simulink model "sim_1_twolink_planar_model"  (R2021a)
settings: Solver=ode15s  StartTime=0.0  StopTime=50  RelTol=1e-5  EnableMultiTasking=on
values from neighbouring files (symbols this model uses):
  b1 = 0.1    [sim_params.m]
  b2 = 0.1    [sim_params.m]
  D = reshape([0.0,0.0,0.0,0.0,0.0,0.0,0.0,0.0],[4,2])    [gen_twolink_ss.m]
  g = 9.80665    [sim_params.m]
  L1x = 0.3    [sim_params.m]
  L1y = 0.050    (= 0.05)    [sim_params.m]
  L1z = 0.05    [sim_params.m]
  L2x = 0.15    [sim_params.m]
  L2y = 0.05    [sim_params.m]
  L2z = 0.05    [sim_params.m]
  m1 = density * L1x*L1y*L1z    (= 2.775)    [sim_params.m]
  m2 = density * L2x*L2y*L2z    (= 1.3875)    [sim_params.m]
  theta1_0 = 0    [sim_params.m]
  theta1_dot_0 = 0    [sim_params.m]
  theta2_0 = 0    [sim_params.m]
  theta2_dot_0 = 0    [sim_params.m]
undefined symbols (not defined in the file or in its folder): X, Y, Z
libraries: sm_lib x11, nesl_utility x10
settings Model: Creator=bhorton  LastModifiedBy=Petronas-Tareq
settings SolverCC: ZeroCrossAlgorithm=Adaptive  AlgebraicLoopSolver=TrustRegion
settings DataIOCC: ReturnWorkspaceOutputs=off
settings OptimizationCC: LifeSpan=inf
settings DebuggingCC: SFUnexpectedBacktrackingDiag=warning  SFNoUnconditionalDefaultTransitionDiag=warning  SFExecutionAtInitializationDiag=none  SFMachineParentedDataDiag=warning  ArithmeticOperatorsInVariantConditions=warning
settings SFSimCC: SimUseLocalCustomCode=off  CustomCodeUndefinedFunction=UseInterfaceOnly
settings RTWCC: RTWUseLocalCustomCode=off
settings CodeAppCC: StateflowObjectComments=on
settings GRTTargetCC: TargetLangStandard=C89/C90 (ANSI)
settings ConfigComp: CovMetricSettings=dw  CovSaveCumulativeToWorkspaceVar=on  CovSaveSingleToWorkspaceVar=on  CovExternalEMLEnable=off
settings SimscapeCC: SimscapeNormalizeSystem=off  SimscapeLogType=all  SimscapeLogDataHistory=10000
settings ExplorerConfigSet: InternalSimMechanicsExplorerSettings="<ExplorerConfiguration><canonicalview>default</canonicalview><AnimationSetting><BasePlaybackSpeed>1.0</BasePlaybackSpeed><PlaybackSpeedFactor>1.0</PlaybackSpeedFactor></AnimationSetting><TilePanel><TileInfo><Tiles Columns=\"1\" Count=\"1\" Rows=\"1\"><Column Weight=\"1\"/><Row Weight=\"1\"/><Tile Height=\"1\" Width=\"1\" X=\"0\" Y=\"0\"/></Tiles></TileInfo><SceneInfo><SceneViewer><BGColor><R>0</R><G>0</G><B>0</B></BGColor><Camera><DoPerspective>off</DoPerspective><Position><X>-0.801082331059953079</X><Y>-0.17844050689426938</Y><Z>1.64033799614712805</Z></Position><Center><X>-0.0582195362274500194</X><Y>-0.543141430318827889</Y><Z>0.0635184868490117349</Z></Center><Up><X>-0.706832108928201031</X><Y>-0.68553501247547266</Y><Z>-0.174442301229848884</Z></Up><ViewLimDist>1</ViewLimDist><YLim>1.1900987998812298</YLim><XLim>2.77184077376740667</XLim></Camera></SceneViewer></SceneInfo></TilePanel><MechEditorPanel><Cameras/><GfxPanelCameraMap/><VideoCreator><PlaybackSpeedRatio>1</PlaybackSpeedRatio><FrameRate>30</FrameRate><VideoFormat>Motion JPEG AVI</VideoFormat><FrameSize>auto</FrameSize></VideoCreator></MechEditorPanel></ExplorerConfiguration>"

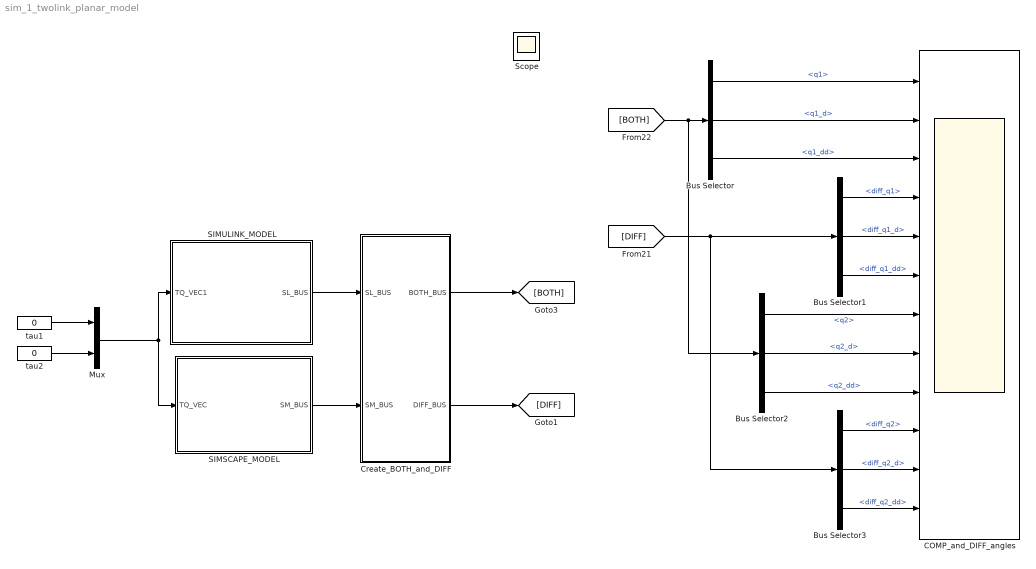
== system sim_1_twolink_planar_model ==
  Bus Selector : BusSelector  OutputSignals=q1,q1_d,q1_dd
  Bus Selector1 : BusSelector  OutputSignals=diff_q1,diff_q1_d,diff_q1_dd
  Bus Selector2 : BusSelector  OutputSignals=q2,q2_d,q2_dd
  Bus Selector3 : BusSelector  OutputSignals=diff_q2,diff_q2_d,diff_q2_dd
  COMP_and_DIFF_angles : Scope  NumInputPorts=12
  Create_BOTH_and_DIFF : Subsystem
  Mux : Mux  Inputs=2
  SIMSCAPE_MODEL : Subsystem
  SIMULINK_MODEL : Subsystem
  tau1 : Constant  Value=0
  tau2 : Constant  Value=0
  Scope : Scope
  wires:
  Mux/1 -> SIMULINK_MODEL/1(TQ_VEC1), SIMSCAPE_MODEL/1(TQ_VEC)
  tau1/1 -> Mux/1
  tau2/1 -> Mux/2
  Bus Selector1/1 -> COMP_and_DIFF_angles/4  "<diff_q1>"
  Bus Selector/3 -> COMP_and_DIFF_angles/3  "<q1_dd>"
  [DIFF] -> Bus Selector1/1, Bus Selector3/1
  Create_BOTH_and_DIFF/1(BOTH_BUS) -> [BOTH]
  Bus Selector1/3 -> COMP_and_DIFF_angles/6  "<diff_q1_dd>"
  SIMULINK_MODEL/1(SL_BUS) -> Create_BOTH_and_DIFF/1(SL_BUS)
  Bus Selector2/2 -> COMP_and_DIFF_angles/8  "<q2_d>"
  Bus Selector1/2 -> COMP_and_DIFF_angles/5  "<diff_q1_d>"
  [BOTH] -> Bus Selector2/1, Bus Selector/1
  Bus Selector2/1 -> COMP_and_DIFF_angles/7  "<q2>"
  Bus Selector3/1 -> COMP_and_DIFF_angles/10  "<diff_q2>"
  Bus Selector2/3 -> COMP_and_DIFF_angles/9  "<q2_dd>"
  Bus Selector/1 -> COMP_and_DIFF_angles/1  "<q1>"
  Bus Selector/2 -> COMP_and_DIFF_angles/2  "<q1_d>"
  Create_BOTH_and_DIFF/2(DIFF_BUS) -> [DIFF]
  Bus Selector3/2 -> COMP_and_DIFF_angles/11  "<diff_q2_d>"
  Bus Selector3/3 -> COMP_and_DIFF_angles/12  "<diff_q2_dd>"
  SIMSCAPE_MODEL/1(SM_BUS) -> Create_BOTH_and_DIFF/2(SM_BUS)

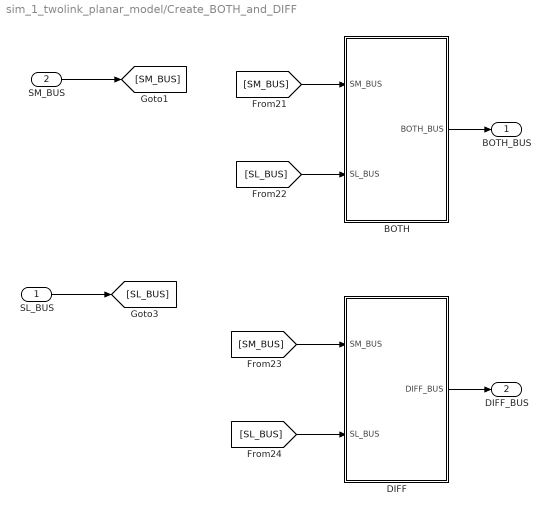
== system sim_1_twolink_planar_model/Create_BOTH_and_DIFF ==
  SL_BUS : Inport
  SM_BUS : Inport  Port=2
  BOTH : Subsystem
  DIFF : Subsystem
  BOTH_BUS : Outport
  DIFF_BUS : Outport  Port=2
  wires:
  SL_BUS/1 -> [SL_BUS]
  SM_BUS/1 -> [SM_BUS]
  [SM_BUS] -> BOTH/1(SM_BUS)
  [SL_BUS] -> BOTH/2(SL_BUS)
  [SM_BUS] -> DIFF/1(SM_BUS)
  [SL_BUS] -> DIFF/2(SL_BUS)
  DIFF/1(DIFF_BUS) -> DIFF_BUS/1
  BOTH/1(BOTH_BUS) -> BOTH_BUS/1

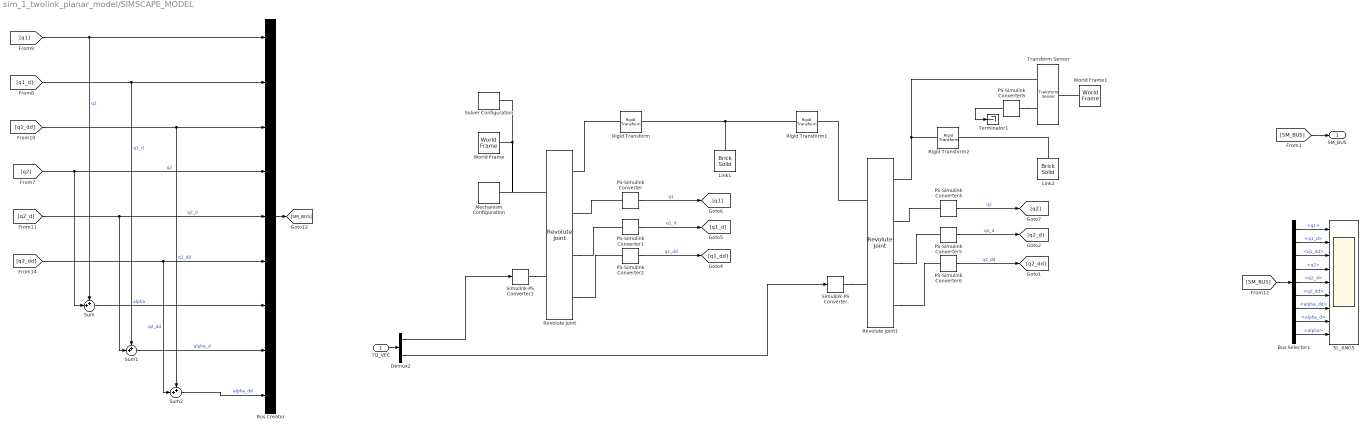
== system sim_1_twolink_planar_model/SIMSCAPE_MODEL ==
  TQ_VEC : Inport
  Bus Creator : BusCreator  Inputs=9
  Bus Selector1 : BusSelector  OutputSignals=q1,q1_d,q1_dd,q2,q2_d,q2_dd,alpha_dd,alpha_d,alpha
  Demux2 : Demux  Outputs=2
  Link1 : sm_lib/Body Elements/Brick Solid  GraphicAmbientColor=[0.15 0.15 0.15 1.0]  BasedOnType=Density  BrickDimensions=[L1x L1y L1z]  BrickDimensionUnits=m  CenterOfMass=[0 0 0]  CenterOfMassUnits=m  GraphicDiffuseColor=[0.8 0.8 1.0]  Density=density  DensityUnits=kg/m^3  DoExposeReferenceFrame=on  GraphicEmissiveColor=[0.0 0.0 0.0 1.0]  ExportEntireGeometry=off  SerializedFrames=<Frames/>  MarkerShape=Sphere  MarkerSize=10  GraphicType=FromGeometry  InertiaType=CalculateFromGeometry  Mass=1  MassUnits=kg  MomentsOfInertia=[1 1 1]  MomentsOfInertiaUnits=kg*m^2  GraphicOpacity=1.0  ProductsOfInertia=[0 0 0]  ProductsOfInertiaUnits=kg*m^2  GraphicShininess=75  GraphicSpecularColor=[0.5 0.5 0.5 1.0]  GraphicVisPropType=SimpleVisualProperties
  Link2 : sm_lib/Body Elements/Brick Solid  GraphicAmbientColor=[0.15 0.15 0.15 1.0]  BasedOnType=Density  BrickDimensions=[L2x L2y L2z]  BrickDimensionUnits=m  CenterOfMass=[0 0 0]  CenterOfMassUnits=m  GraphicDiffuseColor=[1.0 0.6 1.0]  Density=density  DensityUnits=kg/m^3  DoExposeReferenceFrame=on  GraphicEmissiveColor=[0.0 0.0 0.0 1.0]  ExportEntireGeometry=off  SerializedFrames=<Frames/>  MarkerShape=Sphere  MarkerSize=10  GraphicType=FromGeometry  InertiaType=CalculateFromGeometry  Mass=1  MassUnits=kg  MomentsOfInertia=[1 1 1]  MomentsOfInertiaUnits=kg*m^2  GraphicOpacity=1.0  ProductsOfInertia=[0 0 0]  ProductsOfInertiaUnits=kg*m^2  GraphicShininess=75  GraphicSpecularColor=[0.5 0.5 0.5 1.0]  GraphicVisPropType=SimpleVisualProperties
  Mechanism Configuration : sm_lib/Utilities/Mechanism Configuration  UniformGravity=Constant  GravityVector=[0 -g 0 ]  GravityVectorUnits=m/s^2  GravityUnits=m/s^2  LinearizationDelta=1e-4  JointModeTransitionNonlinearIterations=2
  PS-Simulink Converter : nesl_utility/PS-Simulink Converter  PhysicalDomain=network_engine_domain  SubClassName=ps_output  LeftPortType=input  RightPortType=output  PseudoPeriodic=off  Frequencies=[]  Unit=rad  AffineConversion=off
      settings: SourceProductBaseCode=PW,SS
  PS-Simulink Converter1 : nesl_utility/PS-Simulink Converter  PhysicalDomain=network_engine_domain  SubClassName=ps_output  LeftPortType=input  RightPortType=output  PseudoPeriodic=off  Frequencies=[]  Unit=rad/s  AffineConversion=off
      settings: SourceProductBaseCode=PW,SS
  PS-Simulink Converter2 : nesl_utility/PS-Simulink Converter  PhysicalDomain=network_engine_domain  SubClassName=ps_output  LeftPortType=input  RightPortType=output  PseudoPeriodic=off  Frequencies=[]  Unit=rad/s^2  AffineConversion=off
      settings: SourceProductBaseCode=PW,SS
  PS-Simulink Converter4 : nesl_utility/PS-Simulink Converter  PhysicalDomain=network_engine_domain  SubClassName=ps_output  LeftPortType=input  RightPortType=output  PseudoPeriodic=off  Frequencies=[]  Unit=rad  AffineConversion=off
      settings: SourceProductBaseCode=PW,SS
  PS-Simulink Converter5 : nesl_utility/PS-Simulink Converter  PhysicalDomain=network_engine_domain  SubClassName=ps_output  LeftPortType=input  RightPortType=output  PseudoPeriodic=off  Frequencies=[]  Unit=rad/s  AffineConversion=off
      settings: SourceProductBaseCode=PW,SS
  PS-Simulink Converter6 : nesl_utility/PS-Simulink Converter  PhysicalDomain=network_engine_domain  SubClassName=ps_output  LeftPortType=input  RightPortType=output  PseudoPeriodic=off  Frequencies=[]  Unit=rad/s^2  AffineConversion=off
      settings: SourceProductBaseCode=PW,SS
  PS-Simulink Converter8 : nesl_utility/PS-Simulink Converter  PhysicalDomain=network_engine_domain  SubClassName=ps_output  LeftPortType=input  RightPortType=output  PseudoPeriodic=off  Frequencies=[]  Unit=1  AffineConversion=off
      settings: SourceProductBaseCode=PW,SS
  Revolute Joint : sm_lib/Joints/Revolute Joint  JointMode=Normal  SenseConstraintForce=off  SenseConstraintForceX=off  SenseConstraintForceY=off  SenseConstraintForceZ=off  SenseConstraintTorque=off  SenseConstraintTorqueX=off  SenseConstraintTorqueY=off  SenseConstraintTorqueZ=off  SenseTotalForce=off  SenseTotalForceX=off  SenseTotalForceY=off  SenseTotalForceZ=off  SenseTotalTorque=off  SenseTotalTorqueX=off  SenseTotalTorqueY=off  SenseTotalTorqueZ=off  CompositeWrenchDir=BaseOnFollower  CompositeWrenchFrame=BaseFrame  EquilibriumPosition=0  EquilibriumPositionUnits=deg  SpringStiffness=0  SpringStiffnessUnits=N*m/deg  DampingCoefficient=b1  DampingCoefficientUnits=N*m/(rad/s)  TorqueActuationMode=InputTorque  MotionActuationMode=ComputedMotion  SensePosition=on  SenseVelocity=on  SenseAcceleration=on  SenseTorqueForce=off  SenseLowerLimitTorqueForce=off  SenseUpperLimitTorqueForce=off  LowerLimitSpecify=off  LowerLimitBound=-90  LowerLimitBoundUnits=deg  LowerLimitStiffness=1e4  LowerLimitStiffnessUnits=N*m/deg  LowerLimitDamping=10  LowerLimitDampingUnits=N*m/(deg/s)  LowerLimitTransitionRegionWidth=0.1  LowerLimitTransitionRegionWidthUnits=deg  UpperLimitSpecify=off  UpperLimitBound=90  UpperLimitBoundUnits=deg  UpperLimitStiffness=1e4  UpperLimitStiffnessUnits=N*m/deg  UpperLimitDamping=10  UpperLimitDampingUnits=N*m/(deg/s)  UpperLimitTransitionRegionWidth=0.1  UpperLimitTransitionRegionWidthUnits=deg  PositionTargetSpecify=on  PositionTargetPriority=Low  PositionTargetValue=theta1_0  PositionTargetValueUnits=rad  VelocityTargetSpecify=on  VelocityTargetPriority=High  VelocityTargetValue=theta1_dot_0  VelocityTargetValueUnits=rad/s
      settings: AttributesFormatString=|
      | %<DampingCoefficient>
      | %<PositionTargetValue>
      | %<VelocityTargetValue>
  Revolute Joint1 : sm_lib/Joints/Revolute Joint  JointMode=Normal  SenseConstraintForce=off  SenseConstraintForceX=off  SenseConstraintForceY=off  SenseConstraintForceZ=off  SenseConstraintTorque=off  SenseConstraintTorqueX=off  SenseConstraintTorqueY=off  SenseConstraintTorqueZ=off  SenseTotalForce=off  SenseTotalForceX=off  SenseTotalForceY=off  SenseTotalForceZ=off  SenseTotalTorque=off  SenseTotalTorqueX=off  SenseTotalTorqueY=off  SenseTotalTorqueZ=off  CompositeWrenchDir=BaseOnFollower  CompositeWrenchFrame=FollowerFrame  EquilibriumPosition=0  EquilibriumPositionUnits=deg  SpringStiffness=0  SpringStiffnessUnits=N*m/deg  DampingCoefficient=b2  DampingCoefficientUnits=N*m/(rad/s)  TorqueActuationMode=InputTorque  MotionActuationMode=ComputedMotion  SensePosition=on  SenseVelocity=on  SenseAcceleration=on  SenseTorqueForce=off  SenseLowerLimitTorqueForce=off  SenseUpperLimitTorqueForce=off  LowerLimitSpecify=off  LowerLimitBound=-90  LowerLimitBoundUnits=deg  LowerLimitStiffness=1e4  LowerLimitStiffnessUnits=N*m/deg  LowerLimitDamping=10  LowerLimitDampingUnits=N*m/(deg/s)  LowerLimitTransitionRegionWidth=0.1  LowerLimitTransitionRegionWidthUnits=deg  UpperLimitSpecify=off  UpperLimitBound=90  UpperLimitBoundUnits=deg  UpperLimitStiffness=1e4  UpperLimitStiffnessUnits=N*m/deg  UpperLimitDamping=10  UpperLimitDampingUnits=N*m/(deg/s)  UpperLimitTransitionRegionWidth=0.1  UpperLimitTransitionRegionWidthUnits=deg  PositionTargetSpecify=on  PositionTargetPriority=Low  PositionTargetValue=theta2_0  PositionTargetValueUnits=rad  VelocityTargetSpecify=on  VelocityTargetPriority=High  VelocityTargetValue=theta2_dot_0  VelocityTargetValueUnits=rad/s
      settings: AttributesFormatString=|
      | %<DampingCoefficient>
      | %<PositionTargetValue>
      | %<VelocityTargetValue>
  Rigid Transform : sm_lib/Frames and Transforms/Rigid Transform  TranslationMethod=StandardAxis  TranslationStandardOffset=L1x/2  TranslationLengthUnit=m  TranslationStandardAxis=+X  TranslationCartesianOffset=[0 0 0]  TranslationROffset=0  TranslationROffsetUnits=m  TranslationZOffset=0  TranslationZOffsetUnits=m  TranslationThetaOffset=0  TranslationThetaOffsetUnits=deg  RotationMethod=None  RotationAngleUnits=deg  RotationStandardAxis=+Z  RotationAngle=0.0  RotationArbitraryAxis=[0 0 1]  FollAlignAxisA=+X  BaseAlignAxisA=+Y  FollAlignAxisB=+Y  BaseAlignAxisB=+Z  RotationSequenceAxes=FollowerAxes  RotationSequence=XYX  RotationSequenceAngles=[0 0 0]  RotationSequenceAnglesUnits=deg  RotationMatrix=[1 0 0; 0 1 0; 0 0 1]
  Rigid Transform1 : sm_lib/Frames and Transforms/Rigid Transform  TranslationMethod=StandardAxis  TranslationStandardOffset=L1x/2  TranslationLengthUnit=m  TranslationStandardAxis=+X  TranslationCartesianOffset=[0 0 0]  TranslationROffset=0  TranslationROffsetUnits=m  TranslationZOffset=0  TranslationZOffsetUnits=m  TranslationThetaOffset=0  TranslationThetaOffsetUnits=deg  RotationMethod=None  RotationAngleUnits=deg  RotationStandardAxis=+Z  RotationAngle=0.0  RotationArbitraryAxis=[0 0 1]  FollAlignAxisA=+X  BaseAlignAxisA=+Y  FollAlignAxisB=+Y  BaseAlignAxisB=+Z  RotationSequenceAxes=FollowerAxes  RotationSequence=XYX  RotationSequenceAngles=[0 0 0]  RotationSequenceAnglesUnits=deg  RotationMatrix=[1 0 0; 0 1 0; 0 0 1]
  Rigid Transform2 : sm_lib/Frames and Transforms/Rigid Transform  TranslationMethod=StandardAxis  TranslationStandardOffset=L2x/2  TranslationLengthUnit=m  TranslationStandardAxis=+X  TranslationCartesianOffset=[0 0 0]  TranslationROffset=0  TranslationROffsetUnits=m  TranslationZOffset=0  TranslationZOffsetUnits=m  TranslationThetaOffset=0  TranslationThetaOffsetUnits=deg  RotationMethod=None  RotationAngleUnits=deg  RotationStandardAxis=+Z  RotationAngle=0.0  RotationArbitraryAxis=[0 0 1]  FollAlignAxisA=+X  BaseAlignAxisA=+Y  FollAlignAxisB=+Y  BaseAlignAxisB=+Z  RotationSequenceAxes=FollowerAxes  RotationSequence=XYX  RotationSequenceAngles=[0 0 0]  RotationSequenceAnglesUnits=deg  RotationMatrix=[1 0 0; 0 1 0; 0 0 1]
  SL_ANGS : Scope  NumInputPorts=9
  Simulink-PS Converter : nesl_utility/Simulink-PS Converter  PhysicalDomain=network_engine_domain  SubClassName=ps_input  LeftPortType=input  RightPortType=output  PseudoPeriodic=off  Frequencies=[]  NoiseDistribution=none  NoiseParameters=[]  Unit=N*m  AffineConversion=off  FilteringAndDerivatives=zero  SimscapeFilterOrder=1  InputFilterTimeConstant=0.001  UdotUserProvided=1
      settings: SourceProductBaseCode=PW,SS
  Simulink-PS Converter1 : nesl_utility/Simulink-PS Converter  PhysicalDomain=network_engine_domain  SubClassName=ps_input  LeftPortType=input  RightPortType=output  PseudoPeriodic=off  Frequencies=[]  NoiseDistribution=none  NoiseParameters=[]  Unit=N*m  AffineConversion=off  FilteringAndDerivatives=zero  SimscapeFilterOrder=1  InputFilterTimeConstant=0.001  UdotUserProvided=1
      settings: SourceProductBaseCode=PW,SS
  Solver Configuration : nesl_utility/Solver Configuration  PhysicalDomain=network_engine_domain  SubClassName=solver  LeftPortType=input  RightPortType=generic  Tones=[]  Harmonics=[]  SimulateNoise=off  Profile=off  UseLocalSampling=off  EnableSwitchedLinearOptims=on  FrequencyDomain=off  UseCCode=off  RelTol=0.001  AbsTol=1e-06  MinStep=1e-09  ToWorkspace=off  RevertToSquareIcSolve=off  NumHomotopyIterations=100  PhasorMode=off  PhasorModeNumHarmonics=1  DoDC=off  ResidualTolerance=1e-09  UseLocalSolver=off  LocalSolverChoice=NE_TRAPEZOIDAL_ADVANCER  LocalSolverSampleTime=0.01  DoFixedCost=off  MaxNonlinIter=3  MaxModeIter=2  ComputeImpulses=off  ImpulseIterations=2  LinearAlgebra=Sparse  EquationFormulation=NE_TIME_EF  DelaysMemoryBudget=1024  AutomaticFiltering=off  FilteringTimeConstant=0.001  PartitionStorageMethod=AS_NEEDED  PartitionMemoryBudget=1024  PartitionMethod=FAST
      settings: SourceProductBaseCode=PW,SS
  Sum : Sum  Inputs=++|
  Sum1 : Sum  Inputs=++|
  Sum2 : Sum  Inputs=++|
  Terminator1 : Terminator
  Transform Sensor : sm_lib/Frames and Transforms/Transform Sensor  MeasurementFrame=World  SenseAngle=off  SenseAxis=off  SenseAngle1=off  SenseAngle2=off  SenseAngle3=off  SenseQ=off  SenseR=on  SenseOmegaX=off  SenseOmegaY=off  SenseOmegaZ=off  SenseOmega1=off  SenseOmega2=off  SenseOmega3=off  SenseQDot=off  SenseRDot=off  SenseAlphaX=off  SenseAlphaY=off  SenseAlphaZ=off  SenseAlpha1=off  SenseAlpha2=off  SenseAlpha3=off  SenseQDDot=off  SenseRDDot=off  SenseX=off  SenseY=off  SenseZ=off  SenseRad=off  SenseAzim=off  SenseDist=off  SenseInc=off  SenseXDot=off  SenseYDot=off  SenseZDot=off  SenseRadDot=off  SenseAzimDot=off  SenseDistDot=off  SenseIncDot=off  SenseXDDot=off  SenseYDDot=off  SenseZDDot=off  SenseRadDDot=off  SenseAzimDDot=off  SenseDistDDot=off  SenseIncDDot=off
  World Frame : sm_lib/Frames and Transforms/World Frame
  World Frame1 : sm_lib/Frames and Transforms/World Frame
  SM_BUS : Outport
  wires:
  PS-Simulink Converter/1 -> [q1]  "q1"
  PS-Simulink Converter2/1 -> [q1_dd]  "q1_dd"
  PS-Simulink Converter1/1 -> [q1_d]  "q1_d"
  [SM_BUS] -> SM_BUS/1
  PS-Simulink Converter4/1 -> [q2]  "q2"
  PS-Simulink Converter6/1 -> [q2_dd]  "q2_dd"
  PS-Simulink Converter5/1 -> [q2_d]  "q2_d"
  TQ_VEC/1 -> Demux2/1
  Demux2/1 -> Simulink-PS Converter1/1
  Demux2/2 -> Simulink-PS Converter/1
  Bus Selector1/8 -> SL_ANGS/8  "<alpha_d>"
  Bus Selector1/2 -> SL_ANGS/2  "<q1_d>"
  Bus Selector1/5 -> SL_ANGS/5  "<q2_d>"
  Bus Selector1/6 -> SL_ANGS/6  "<q2_dd>"
  Bus Selector1/1 -> SL_ANGS/1  "<q1>"
  Bus Selector1/9 -> SL_ANGS/9  "<alpha>"
  Bus Selector1/7 -> SL_ANGS/7  "<alpha_dd>"
  Bus Selector1/3 -> SL_ANGS/3  "<q1_dd>"
  Sum1/1 -> Bus Creator/8  "alpha_d"
  [q1_dd] -> Bus Creator/3, Sum2/1  "q1_dd"
  [q1] -> Sum/1, Bus Creator/1  "q1"
  Sum/1 -> Bus Creator/7  "alpha"
  [q2] -> Sum/2, Bus Creator/4  "q2"
  [q2_d] -> Sum1/2, Bus Creator/5  "q2_d"
  Bus Creator/1 -> [SM_BUS]
  [q1_d] -> Sum1/1, Bus Creator/2  "q1_d"
  Sum2/1 -> Bus Creator/9  "alpha_dd"
  [SM_BUS] -> Bus Selector1/1
  [q2_dd] -> Sum2/2, Bus Creator/6  "q2_dd"
  Bus Selector1/4 -> SL_ANGS/4  "<q2>"
  PS-Simulink Converter8/1 -> Terminator1/1
  connections:
  World Frame/RConn1 -- Revolute Joint/LConn1 -- Mechanism Configuration/RConn1 -- Solver Configuration/RConn1
  Rigid Transform1/LConn1 -- Link1/RConn1 -- Rigid Transform/RConn1
  Revolute Joint/RConn3 -- PS-Simulink Converter1/LConn1
  Revolute Joint/RConn4 -- PS-Simulink Converter2/LConn1
  Rigid Transform/LConn1 -- Revolute Joint/RConn1
  PS-Simulink Converter/LConn1 -- Revolute Joint/RConn2
  Revolute Joint1/LConn1 -- Rigid Transform1/RConn1
  Revolute Joint1/RConn3 -- PS-Simulink Converter5/LConn1
  Revolute Joint1/RConn2 -- PS-Simulink Converter4/LConn1
  Revolute Joint1/RConn4 -- PS-Simulink Converter6/LConn1
  Link2/RConn1 -- Rigid Transform2/RConn1
  Rigid Transform2/LConn1 -- Transform Sensor/RConn1 -- Revolute Joint1/RConn1
  World Frame1/RConn1 -- Transform Sensor/LConn1
  PS-Simulink Converter8/LConn1 -- Transform Sensor/RConn2
  Simulink-PS Converter/RConn1 -- Revolute Joint1/LConn2
  Simulink-PS Converter1/RConn1 -- Revolute Joint/LConn2

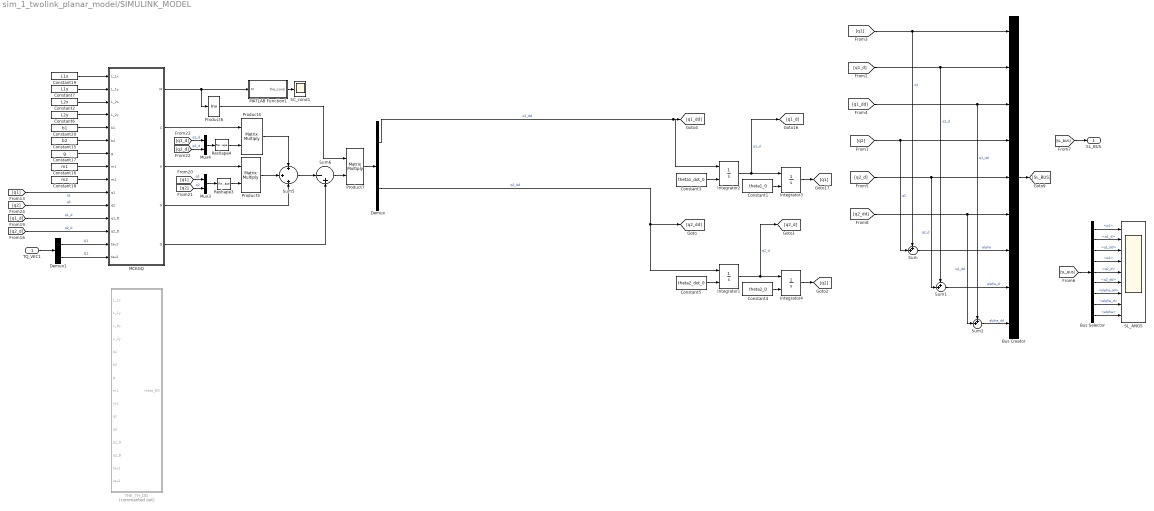
== system sim_1_twolink_planar_model/SIMULINK_MODEL ==
  TQ_VEC1 : Inport
  Bus Creator : BusCreator  Inputs=9
  Bus Selector : BusSelector  OutputSignals=q1,q1_d,q1_dd,q2,q2_d,q2_dd,alpha_dd,alpha_d,alpha
  Constant1 : Constant  Value=theta1_0
  Constant15 : Constant  Value=b2
  Constant16 : Constant  Value=m1
  Constant17 : Constant  Value=g
  Constant18 : Constant  Value=m2
  Constant19 : Constant  Value=L1x
  Constant2 : Constant  Value=L2x
  Constant20 : Constant  Value=b1
  Constant3 : Constant  Value=theta1_dot_0
  Constant4 : Constant  Value=theta2_0
  Constant5 : Constant  Value=theta2_dot_0
  Constant6 : Constant  Value=L2y
  Constant7 : Constant  Value=L1y
  Demux : Demux  Outputs=2
  Demux1 : Demux  Outputs=2
  Integrator{1..4} (4 alike) : Integrator  InitialConditionSource=external
  MATLAB Function1 : MATLAB Function  TreatAsAtomicUnit=on
  MCKGQ : MATLAB Function  TreatAsAtomicUnit=on
  Mux3 : Mux  Inputs=2
  Mux4 : Mux  Inputs=2
  Product4 : Product  Multiplication=Matrix(*)
  Product5 : Product  Multiplication=Matrix(*)
  Product6 : Product  Inputs=/  Multiplication=Matrix(*)
  Product7 : Product  Multiplication=Matrix(*)
  Reshape3 : Reshape  OutputDimensionality=Column vector (2-D)
  Reshape4 : Reshape  OutputDimensionality=Column vector (2-D)
  SC_cond1 : Scope
  SL_ANGS : Scope  NumInputPorts=9
  Sum : Sum  Inputs=++|
  Sum1 : Sum  Inputs=++|
  Sum2 : Sum  Inputs=++|
  Sum5 : Sum  Inputs=+|+|+
  Sum6 : Sum  Inputs=|-+
  THE_TH_DD : MATLAB Function  Commented=on  TreatAsAtomicUnit=on
  SL_BUS : Outport
  wires:
  [SL_BUS] -> Bus Selector/1
  [SL_BUS] -> SL_BUS/1
  Bus Selector/2 -> SL_ANGS/2  "<q1_d>"
  Bus Selector/3 -> SL_ANGS/3  "<q1_dd>"
  Bus Selector/1 -> SL_ANGS/1  "<q1>"
  Bus Selector/4 -> SL_ANGS/4  "<q2>"
  Bus Selector/5 -> SL_ANGS/5  "<q2_d>"
  Bus Selector/6 -> SL_ANGS/6  "<q2_dd>"
  Bus Selector/7 -> SL_ANGS/7  "<alpha_dd>"
  Bus Selector/8 -> SL_ANGS/8  "<alpha_d>"
  Bus Selector/9 -> SL_ANGS/9  "<alpha>"
  Integrator3/1 -> [q1]
  Integrator2/1 -> [q1_d], Integrator3/1  "q1_d"
  Constant3/1 -> Integrator2/2
  Constant1/1 -> Integrator3/2
  Integrator1/1 -> [q2_d], Integrator4/1  "q2_d"
  Constant4/1 -> Integrator4/2
  Integrator4/1 -> [q2]
  Constant5/1 -> Integrator1/2
  Sum2/1 -> Bus Creator/9  "alpha_dd"
  [q1_d] -> Sum1/1, Bus Creator/2  "q1_d"
  [q2_d] -> Sum1/2, Bus Creator/5  "q2_d"
  Bus Creator/1 -> [SL_BUS]
  [q2] -> Sum/2, Bus Creator/4  "q2"
  [q2_dd] -> Sum2/2, Bus Creator/6  "q2_dd"
  [q1] -> Bus Creator/1, Sum/1  "q1"
  Sum1/1 -> Bus Creator/8  "alpha_d"
  [q1_dd] -> Bus Creator/3, Sum2/1  "q1_dd"
  Sum/1 -> Bus Creator/7  "alpha"
  Demux/1 -> Integrator2/1, [q1_dd]  "q1_dd"
  Demux/2 -> Integrator1/1, [q2_dd]  "q2_dd"
  MCKGQ/5(Q) -> Sum6/2
  [q1] -> Mux3/1  "q1"
  Sum6/1 -> Product7/2
  [q2] -> Mux3/2  "q2"
  Sum5/1 -> Sum6/1
  Product4/1 -> Sum5/1
  Constant18/1 -> MCKGQ/9(m2)
  Product5/1 -> Sum5/2
  Demux1/2 -> MCKGQ/15(tau2)  "Q2"
  MCKGQ/3(K) -> Product5/1
  MATLAB Function1/1(the_cond) -> SC_cond1/1
  Product6/1 -> Product7/1
  Constant20/1 -> MCKGQ/5(b1)
  Reshape3/1 -> Product5/2
  [q1] -> MCKGQ/10(q1)  "q1"
  Constant6/1 -> MCKGQ/4(L_2y)
  MCKGQ/4(G) -> Sum5/3
  Constant15/1 -> MCKGQ/6(b2)
  [q1_d] -> MCKGQ/12(q1_D)  "q1_d"
  Constant2/1 -> MCKGQ/3(L_2x)
  Constant19/1 -> MCKGQ/1(L_1x)
  Constant7/1 -> MCKGQ/2(L_1y)
  MCKGQ/2(C) -> Product4/1
  [q1_d] -> Mux4/1  "q1_d"
  Mux3/1 -> Reshape3/1
  Reshape4/1 -> Product4/2
  [q2_d] -> MCKGQ/13(q2_D)  "q2_d"
  [q2_d] -> Mux4/2  "q2_d"
  Demux1/1 -> MCKGQ/14(tau1)  "Q1"
  MCKGQ/1(M) -> MATLAB Function1/1(M), Product6/1
  Mux4/1 -> Reshape4/1
  [q2] -> MCKGQ/11(q2)  "q2"
  Constant17/1 -> MCKGQ/7(g)
  Constant16/1 -> MCKGQ/8(m1)
  TQ_VEC1/1 -> Demux1/1
  Product7/1 -> Demux/1

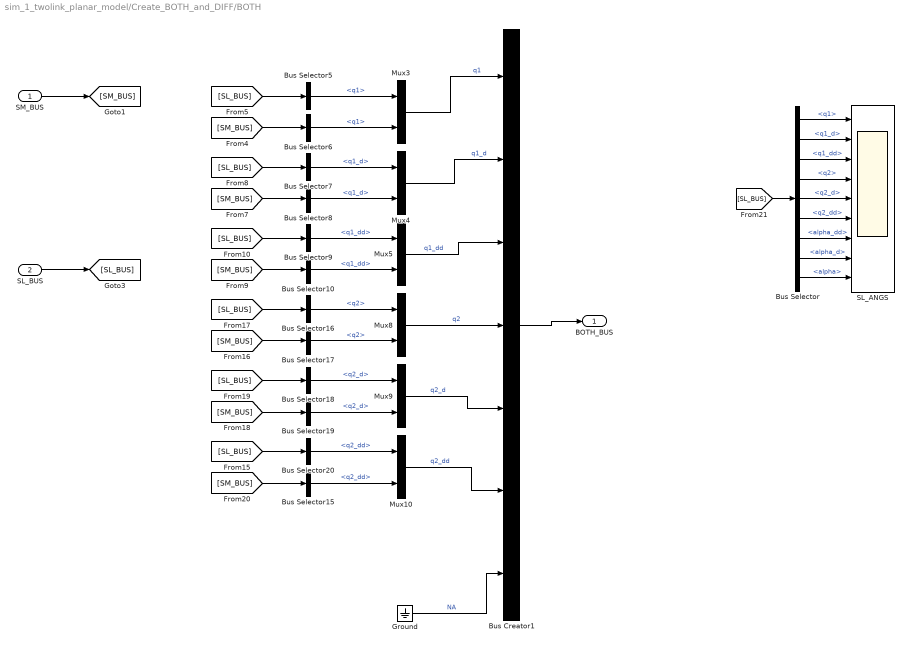
== system sim_1_twolink_planar_model/Create_BOTH_and_DIFF/BOTH ==
  SM_BUS : Inport
  SL_BUS : Inport  Port=2
  Bus Creator1 : BusCreator  Inputs=7
  Bus Selector : BusSelector  OutputSignals=q1,q1_d,q1_dd,q2,q2_d,q2_dd,alpha_dd,alpha_d,alpha
  Bus Selector10 : BusSelector  OutputSignals=q1_dd
  Bus Selector15 : BusSelector  OutputSignals=q2_dd
  Bus Selector16 : BusSelector  OutputSignals=q2
  Bus Selector17 : BusSelector  OutputSignals=q2
  Bus Selector18 : BusSelector  OutputSignals=q2_d
  Bus Selector19 : BusSelector  OutputSignals=q2_d
  Bus Selector20 : BusSelector  OutputSignals=q2_dd
  Bus Selector5 : BusSelector  OutputSignals=q1
  Bus Selector6 : BusSelector  OutputSignals=q1
  Bus Selector7 : BusSelector  OutputSignals=q1_d
  Bus Selector8 : BusSelector  OutputSignals=q1_d
  Bus Selector9 : BusSelector  OutputSignals=q1_dd
  Ground : Ground
  Mux{3..5,8..10} (6 alike) : Mux  Inputs=2
  SL_ANGS : Scope  NumInputPorts=9
  BOTH_BUS : Outport
  wires:
  SL_BUS/1 -> [SL_BUS]
  SM_BUS/1 -> [SM_BUS]
  [SM_BUS] -> Bus Selector6/1
  [SL_BUS] -> Bus Selector5/1
  [SL_BUS] -> Bus Selector7/1
  [SM_BUS] -> Bus Selector8/1
  [SL_BUS] -> Bus Selector9/1
  [SM_BUS] -> Bus Selector10/1
  Bus Selector5/1 -> Mux3/1  "<q1>"
  Bus Selector6/1 -> Mux3/2  "<q1>"
  Bus Selector7/1 -> Mux4/1  "<q1_d>"
  Bus Selector8/1 -> Mux4/2  "<q1_d>"
  Bus Selector9/1 -> Mux5/1  "<q1_dd>"
  Bus Selector10/1 -> Mux5/2  "<q1_dd>"
  Mux3/1 -> Bus Creator1/1  "q1"
  Mux4/1 -> Bus Creator1/2  "q1_d"
  Mux5/1 -> Bus Creator1/3  "q1_dd"
  [SM_BUS] -> Bus Selector17/1
  [SL_BUS] -> Bus Selector16/1
  [SL_BUS] -> Bus Selector18/1
  [SM_BUS] -> Bus Selector19/1
  [SL_BUS] -> Bus Selector20/1
  [SM_BUS] -> Bus Selector15/1
  Bus Selector16/1 -> Mux8/1  "<q2>"
  Bus Selector17/1 -> Mux8/2  "<q2>"
  Bus Selector18/1 -> Mux9/1  "<q2_d>"
  Bus Selector19/1 -> Mux9/2  "<q2_d>"
  Bus Selector20/1 -> Mux10/1  "<q2_dd>"
  Bus Selector15/1 -> Mux10/2  "<q2_dd>"
  Mux8/1 -> Bus Creator1/4  "q2"
  Mux9/1 -> Bus Creator1/5  "q2_d"
  Mux10/1 -> Bus Creator1/6  "q2_dd"
  Ground/1 -> Bus Creator1/7  "NA"
  Bus Selector/8 -> SL_ANGS/8  "<alpha_d>"
  Bus Selector/2 -> SL_ANGS/2  "<q1_d>"
  Bus Selector/9 -> SL_ANGS/9  "<alpha>"
  Bus Selector/6 -> SL_ANGS/6  "<q2_dd>"
  Bus Selector/3 -> SL_ANGS/3  "<q1_dd>"
  Bus Selector/7 -> SL_ANGS/7  "<alpha_dd>"
  [SL_BUS] -> Bus Selector/1
  Bus Selector/1 -> SL_ANGS/1  "<q1>"
  Bus Selector/5 -> SL_ANGS/5  "<q2_d>"
  Bus Selector/4 -> SL_ANGS/4  "<q2>"
  Bus Creator1/1 -> BOTH_BUS/1

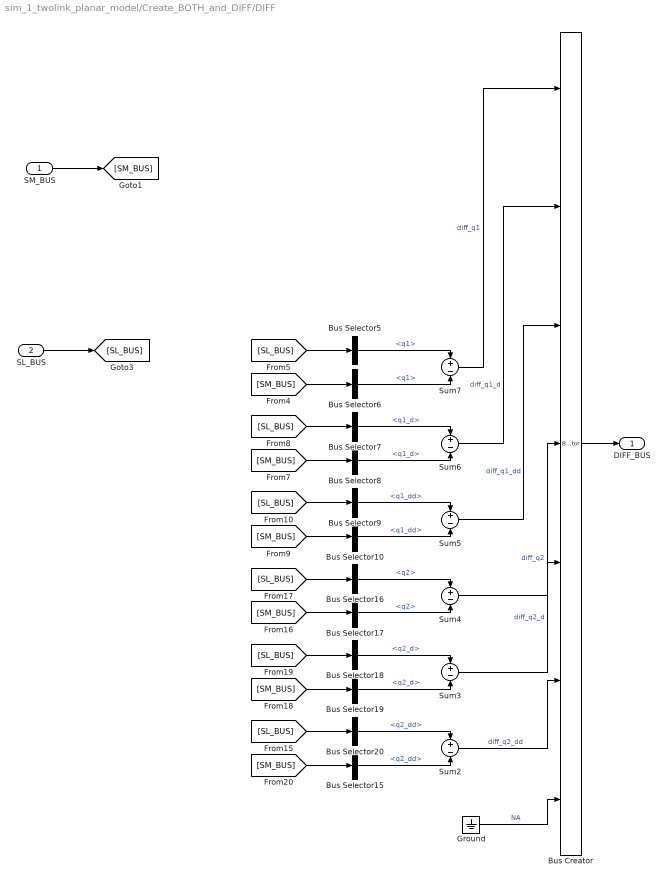
== system sim_1_twolink_planar_model/Create_BOTH_and_DIFF/DIFF ==
  SM_BUS : Inport
  SL_BUS : Inport  Port=2
  Bus Creator : BusCreator  Inputs=7
  Bus Selector10 : BusSelector  OutputSignals=q1_dd
  Bus Selector15 : BusSelector  OutputSignals=q2_dd
  Bus Selector16 : BusSelector  OutputSignals=q2
  Bus Selector17 : BusSelector  OutputSignals=q2
  Bus Selector18 : BusSelector  OutputSignals=q2_d
  Bus Selector19 : BusSelector  OutputSignals=q2_d
  Bus Selector20 : BusSelector  OutputSignals=q2_dd
  Bus Selector5 : BusSelector  OutputSignals=q1
  Bus Selector6 : BusSelector  OutputSignals=q1
  Bus Selector7 : BusSelector  OutputSignals=q1_d
  Bus Selector8 : BusSelector  OutputSignals=q1_d
  Bus Selector9 : BusSelector  OutputSignals=q1_dd
  Ground : Ground
  Sum{2..7} (6 alike) : Sum  Inputs=+|-
  DIFF_BUS : Outport
  wires:
  SL_BUS/1 -> [SL_BUS]
  SM_BUS/1 -> [SM_BUS]
  [SM_BUS] -> Bus Selector6/1
  [SL_BUS] -> Bus Selector5/1
  [SL_BUS] -> Bus Selector7/1
  [SM_BUS] -> Bus Selector8/1
  [SL_BUS] -> Bus Selector9/1
  [SM_BUS] -> Bus Selector10/1
  Bus Selector5/1 -> Sum7/1  "<q1>"
  Bus Selector6/1 -> Sum7/2  "<q1>"
  Bus Selector7/1 -> Sum6/1  "<q1_d>"
  Bus Selector8/1 -> Sum6/2  "<q1_d>"
  Bus Selector9/1 -> Sum5/1  "<q1_dd>"
  Bus Selector10/1 -> Sum5/2  "<q1_dd>"
  Sum7/1 -> Bus Creator/1  "diff_q1"
  Sum6/1 -> Bus Creator/2  "diff_q1_d"
  Bus Creator/1 -> DIFF_BUS/1
  Sum5/1 -> Bus Creator/3  "diff_q1_dd"
  [SM_BUS] -> Bus Selector17/1
  [SL_BUS] -> Bus Selector16/1
  [SL_BUS] -> Bus Selector18/1
  [SM_BUS] -> Bus Selector19/1
  [SL_BUS] -> Bus Selector20/1
  [SM_BUS] -> Bus Selector15/1
  Bus Selector16/1 -> Sum4/1  "<q2>"
  Bus Selector17/1 -> Sum4/2  "<q2>"
  Bus Selector18/1 -> Sum3/1  "<q2_d>"
  Bus Selector19/1 -> Sum3/2  "<q2_d>"
  Bus Selector20/1 -> Sum2/1  "<q2_dd>"
  Bus Selector15/1 -> Sum2/2  "<q2_dd>"
  Sum4/1 -> Bus Creator/4  "diff_q2"
  Sum3/1 -> Bus Creator/5  "diff_q2_d"
  Sum2/1 -> Bus Creator/6  "diff_q2_dd"
  Ground/1 -> Bus Creator/7  "NA"

== matlab function sim_1_twolink_planar_model/SIMULINK_MODEL/THE_TH_DD ==
  data: L_1x input; theta_DD output; L_1y input; L_2x input; L_2y input; b1 input; b2 input; g input; m1 input; m2 input; q1 input; q2 input; q1_D input; q2_D input; tau1 input; tau2 input
function theta_DD = THE_TH_DD(L_1x,L_1y,L_2x,L_2y,b1,b2,g,m1,m2,q1,q2,q1_D,q2_D,tau1,tau2)
%#codegen

%    This function was generated by the Symbolic Math Toolbox version 8.7.
%    30-May-2022 13:59:37

et1 = (L_1x.^2.*m1.*4.0+L_1x.^2.*m2.*1.2e+1+L_1y.^2.*m1+L_2x.^2.*m2.*3.0+L_1x.*L_2x.*m2.*cos(q2).*1.2e+1).*(-tau2+b2.*q2_D+(L_1x.*L_2x.*m2.*q1_D.^2.*sin(q2))./2.0+(L_2x.*g.*m2.*cos(q1).*cos(q2))./2.0-(L_2x.*g.*m2.*sin(q1).*sin(q2))./2.0);
et2 = -1.2e+1./(L_2x.^4.*m2.^2.*3.0+L_1x.^2.*L_2x.^2.*m2.^2.*4.8e+1+L_1x.^2.*L_2y.^2.*m2.^2.*1.2e+1+L_2x.^2.*L_2y.^2.*m2.^2.*3.0+L_1x.^2.*L_2x.^2.*m1.*m2.*1.6e+1+L_1x.^2.*L_2y.^2.*m1.*m2.*4.0+L_1y.^2.*L_2x.^2.*m1.*m2.*4.0+L_1y.^2.*L_2y.^2.*m1.*m2-L_1x.^2.*L_2x.^2.*m2.^2.*cos(q2).^2.*3.6e+1+L_1x.*L_2x.^3.*m2.^2.*cos(q2).*1.2e+1+L_1x.*L_2x.*L_2y.^2.*m2.^2.*cos(q2).*1.2e+1);
et3 = ((L_2x.^2+L_1x.*L_2x.*cos(q2).*2.0).*(-tau2+b2.*q2_D+(L_1x.*L_2x.*m2.*q1_D.^2.*sin(q2))./2.0+(L_2x.*g.*m2.*cos(q1).*cos(q2))./2.0-(L_2x.*g.*m2.*sin(q1).*sin(q2))./2.0).*3.6e+1)./(L_2x.^4.*m2.*3.0+L_1x.^2.*L_2x.^2.*m1.*1.6e+1+L_1x.^2.*L_2x.^2.*m2.*4.8e+1+L_1x.^2.*L_2y.^2.*m1.*4.0+L_1y.^2.*L_2x.^2.*m1.*4.0+L_1x.^2.*L_2y.^2.*m2.*1.2e+1+L_1y.^2.*L_2y.^2.*m1+L_2x.^2.*L_2y.^2.*m2.*3.0-L_1x.^2.*L_2x.^2.*m2.*cos(q2).^2.*3.6e+1+L_1x.*L_2x.^3.*m2.*cos(q2).*1.2e+1+L_1x.*L_2x.*L_2y.^2.*m2.*cos(q2).*1.2e+1);
et4 = ((L_2x.^2.*4.0+L_2y.^2).*(tau1-b1.*q1_D-(L_1x.*g.*m1.*cos(q1))./2.0-L_1x.*g.*m2.*cos(q1)+(L_1x.*L_2x.*m2.*q2_D.^2.*sin(q2))./2.0-(L_2x.*g.*m2.*cos(q1).*cos(q2))./2.0+(L_2x.*g.*m2.*sin(q1).*sin(q2))./2.0+L_1x.*L_2x.*m2.*q1_D.*q2_D.*sin(q2)).*1.2e+1)./(L_2x.^4.*m2.*3.0+L_1x.^2.*L_2x.^2.*m1.*1.6e+1+L_1x.^2.*L_2x.^2.*m2.*4.8e+1+L_1x.^2.*L_2y.^2.*m1.*4.0+L_1y.^2.*L_2x.^2.*m1.*4.0+L_1x.^2.*L_2y.^2.*m2.*1.2e+1+L_1y.^2.*L_2y.^2.*m1+L_2x.^2.*L_2y.^2.*m2.*3.0-L_1x.^2.*L_2x.^2.*m2.*cos(q2).^2.*3.6e+1+L_1x.*L_2x.^3.*m2.*cos(q2).*1.2e+1+L_1x.*L_2x.*L_2y.^2.*m2.*cos(q2).*1.2e+1);
theta_DD = [et3+et4;et1.*et2-((L_2x.^2+L_1x.*L_2x.*cos(q2).*2.0).*(tau1-b1.*q1_D-(L_1x.*g.*m1.*cos(q1))./2.0-L_1x.*g.*m2.*cos(q1)+(L_1x.*L_2x.*m2.*q2_D.^2.*sin(q2))./2.0-(L_2x.*g.*m2.*cos(q1).*cos(q2))./2.0+(L_2x.*g.*m2.*sin(q1).*sin(q2))./2.0+L_1x.*L_2x.*m2.*q1_D.*q2_D.*sin(q2)).*3.6e+1)./(L_2x.^4.*m2.*3.0+L_1x.^2.*L_2x.^2.*m1.*1.6e+1+L_1x.^2.*L_2x.^2.*m2.*4.8e+1+L_1x.^2.*L_2y.^2.*m1.*4.0+L_1y.^2.*L_2x.^2.*m1.*4.0+L_1x.^2.*L_2y.^2.*m2.*1.2e+1+L_1y.^2.*L_2y.^2.*m1+L_2x.^2.*L_2y.^2.*m2.*3.0-L_1x.^2.*L_2x.^2.*m2.*cos(q2).^2.*3.6e+1+L_1x.*L_2x.^3.*m2.*cos(q2).*1.2e+1+L_1x.*L_2x.*L_2y.^2.*m2.*cos(q2).*1.2e+1)];

== matlab function sim_1_twolink_planar_model/SIMULINK_MODEL/MCKGQ ==
  data: L_1x input; M output; L_1y input; L_2x input; L_2y input; b1 input; b2 input; g input; m1 input; m2 input; q1 input; q2 input; q1_D input; q2_D input; tau1 input; tau2 input; C output; K output; G output; Q output
function [M,C,K,G,Q] = MCKGQ(L_1x,L_1y,L_2x,L_2y,b1,b2,g,m1,m2,q1,q2,q1_D,q2_D,tau1,tau2)
%#codegen

%    This function was generated by the Symbolic Math Toolbox version 8.7.
%    30-May-2022 13:59:37

M = reshape([(L_1x.^2.*m1)./3.0+L_1x.^2.*m2+(L_1y.^2.*m1)./1.2e+1+(L_2x.^2.*m2)./4.0+L_1x.*L_2x.*m2.*cos(q2),(L_2x.*m2.*(L_2x+L_1x.*cos(q2).*2.0))./4.0,(L_2x.*m2.*(L_2x+L_1x.*cos(q2).*2.0))./4.0,(m2.*(L_2x.^2.*4.0+L_2y.^2))./1.2e+1],[2,2]);
if nargout > 1
    C = reshape([-L_1x.*L_2x.*m2.*q2_D.*sin(q2),(L_1x.*L_2x.*m2.*q1_D.*sin(q2))./2.0,L_1x.*L_2x.*m2.*q2_D.*sin(q2).*(-1.0./2.0),0.0],[2,2]);
end
if nargout > 2
    K = reshape([0.0,0.0,0.0,0.0],[2,2]);
end
if nargout > 3
    G = [(g.*(L_2x.*m2.*cos(q1+q2)+L_1x.*m1.*cos(q1)+L_1x.*m2.*cos(q1).*2.0))./2.0;(L_2x.*g.*m2.*cos(q1+q2))./2.0];
end
if nargout > 4
    Q = [tau1-b1.*q1_D;tau2-b2.*q2_D];
end

== matlab function sim_1_twolink_planar_model/SIMULINK_MODEL/MATLAB Function1 ==
  data: M input; the_cond output
function the_cond = COND(M)
%#codegen

the_cond = cond(M);

end
